simulink model "CCCV_Trial_6"  (R2022b)
settings: Solver=VariableStepAuto  StartTime=0.0  StopTime=3600  RelTol=1e-3
libraries: spsSeriesRLCBranchLib x7, spsCurrentMeasurementLib x2, spsDCVoltageSourceLib x1, spsDiodeLib x1, spsGroundLib x1, spsMosfetLib x1, spsVoltageMeasurementLib x1, sps_lib x1
settings Model: Creator=Haposan  LastModifiedBy=Haposan

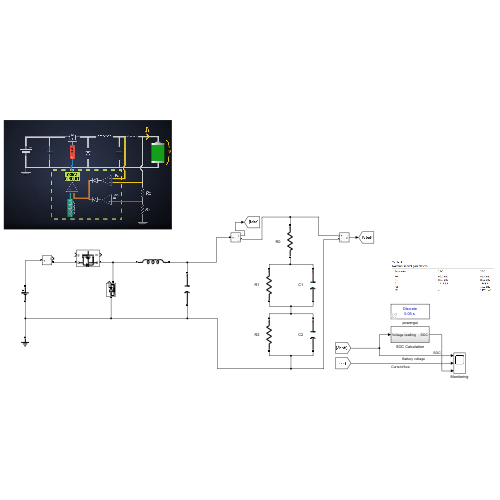
[thumbnail: Simulink's stored preview of the top-level diagram]
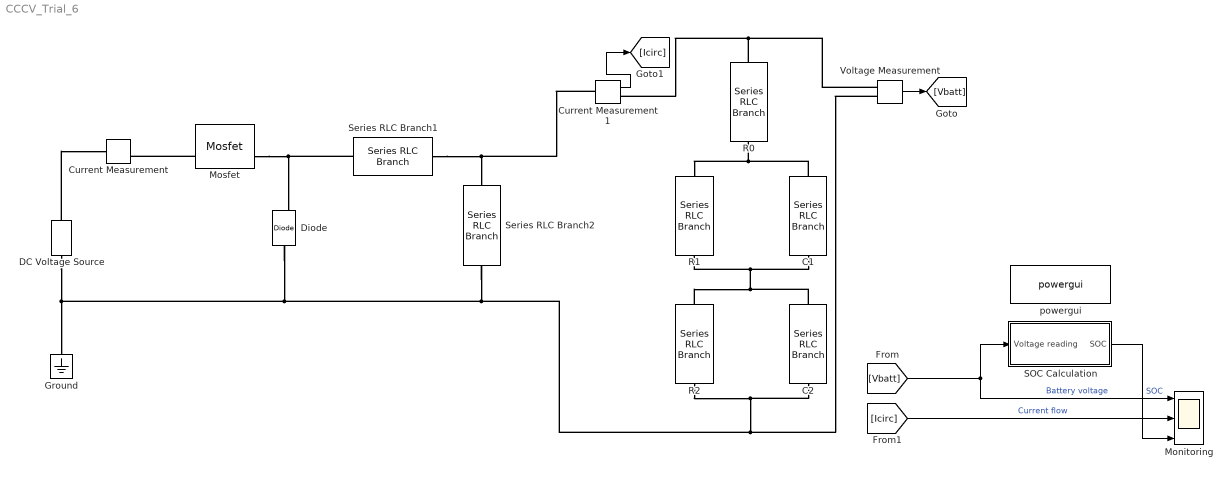
== system CCCV_Trial_6 ==
  C1 : spsSeriesRLCBranchLib/Series RLC Branch  LConnTagsString=__new0  RConnTagsString=__new0  BranchType=C  Resistance=1  Inductance=1e-3  SetiL0=off  InitialCurrent=0  Capacitance=1148  Setx0=off  InitialVoltage=0  Measurements=None
  C2 : spsSeriesRLCBranchLib/Series RLC Branch  LConnTagsString=__new0  RConnTagsString=__new0  BranchType=C  Resistance=1  Inductance=1e-3  SetiL0=off  InitialCurrent=0  Capacitance=117.1e-3  Setx0=off  InitialVoltage=0  Measurements=None
  Current Measurement : spsCurrentMeasurementLib/Current Measurement  PhasorSimulation=off  OutputType=Complex  PSBequivalent=0
  Current Measurement1 : spsCurrentMeasurementLib/Current Measurement  PhasorSimulation=off  OutputType=Complex  PSBequivalent=0
  DC Voltage Source : spsDCVoltageSourceLib/DC Voltage Source  Amplitude=4.2  Measurements=None
  Diode : spsDiodeLib/Diode  Ron=0.001  Lon=0  Vf=0.8  IC=0  UseSnubber=0  Rs=500  Cs=250e-9  Measurements=on
  Ground : spsGroundLib/Ground  LConnTagsString=a
  Monitoring : Scope  NumInputPorts=3
  Mosfet : spsMosfetLib/Mosfet  Ron=0.1  Lon=0  Rd=0.01  Vfd=0  IC=0  Rs=1e5  Cs=inf  Measurements=on
  R0 : spsSeriesRLCBranchLib/Series RLC Branch  LConnTagsString=__new0  RConnTagsString=__new0  BranchType=R  Resistance=56.4e-3  Inductance=1e-3  SetiL0=off  InitialCurrent=0  Capacitance=200e-6  Setx0=off  InitialVoltage=0  Measurements=None
  R1 : spsSeriesRLCBranchLib/Series RLC Branch  LConnTagsString=__new0  RConnTagsString=__new0  BranchType=R  Resistance=35.2e-3  Inductance=1e-3  SetiL0=off  InitialCurrent=0  Capacitance=200e-6  Setx0=off  InitialVoltage=0  Measurements=None
  R2 : spsSeriesRLCBranchLib/Series RLC Branch  LConnTagsString=__new0  RConnTagsString=__new0  BranchType=R  Resistance=13.2e-3  Inductance=1e-3  SetiL0=off  InitialCurrent=0  Capacitance=200e-6  Setx0=off  InitialVoltage=0  Measurements=None
  SOC Calculation : Subsystem
  Series RLC Branch1 : spsSeriesRLCBranchLib/Series RLC Branch  LConnTagsString=__new0  RConnTagsString=__new0  BranchType=L  Resistance=1  Inductance=150e-4  SetiL0=off  InitialCurrent=0  Capacitance=1e-6  Setx0=off  InitialVoltage=0  Measurements=None
  Series RLC Branch2 : spsSeriesRLCBranchLib/Series RLC Branch  LConnTagsString=__new0  RConnTagsString=__new0  BranchType=C  Resistance=1  Inductance=1e-3  SetiL0=off  InitialCurrent=0  Capacitance=1  Setx0=off  InitialVoltage=0  Measurements=None
  Voltage Measurement : spsVoltageMeasurementLib/Voltage Measurement  PhasorSimulation=off  OutputType=Complex  PSBequivalent=0
  powergui : sps_lib/powergui  Priority=1  SimulationMode=Discrete  SampleTime=50e-3  frequency=60  Iterations=50  frequencyindice=0  Pbase=100e6  ErrMax=1e-4  UnitsV=kV  UnitsW=MW  buscounter=0  FunctionMessages=off  echomessages=off  EnableUseOfTLC=off  CurrentSourceSwitches=off  DisableSnubberDevices=off  DisableRonSwitches=off  DisableVfSwitches=off  DisplayEquations=off  AutomaticDiscreteSolvers=off  SolverType=Tustin/Backward Euler (TBE)  Interpol=off  ExternalGateDelay=off  methode=off  Ts=100  x0status=blocks  SPID=on  SwTol=0  HookPort=off  NonlinearTolerance=1e-4  nMaxIteration=100  ContinueOnMaxIteration=off  RestoreLinks=warning  ResistiveCurrentMeasurement=off  Frange=[0:2:500]  Ylog=off  Xlog=on  ShowGrid=off  save=off  variable=ZData  structure=0  ZoomFFT=off  StartTime=0.0  cycles=1  DisplayStyle=1  fundamental=60  FreqAxis=off  MaxFrequency=1000  frequencyindicesteady=1  RmsSteady=1  display=off
  wires:
  SOC Calculation/1(SOC) -> Monitoring/3  "SOC"
  [Icirc] -> Monitoring/2  "Current flow"
  [Vbatt] -> SOC Calculation/1(Voltage reading), Monitoring/1  "Battery voltage"
  Voltage Measurement/1 -> [Vbatt]
  Current Measurement1/1 -> [Icirc]
  connections:
  DC Voltage Source/RConn1 -- Current Measurement/LConn1
  DC Voltage Source/LConn1 -- Voltage Measurement/LConn2 -- C2/RConn1 -- R2/RConn1 -- Series RLC Branch2/RConn1 -- Diode/LConn1 -- Ground/LConn1
  Series RLC Branch1/RConn1 -- Mosfet/RConn1 -- Diode/RConn1
  Series RLC Branch1/LConn1 -- Current Measurement1/LConn1 -- Series RLC Branch2/LConn1
  C1/LConn1 -- R1/LConn1 -- R0/RConn1
  C2/LConn1 -- R2/LConn1 -- C1/RConn1 -- R1/RConn1
  R0/LConn1 -- Voltage Measurement/LConn1 -- Current Measurement1/RConn1
  Mosfet/LConn1 -- Current Measurement/RConn1

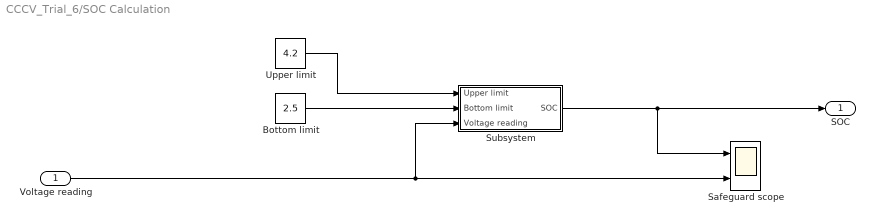
== system CCCV_Trial_6/SOC Calculation ==
  Voltage reading : Inport
  Bottom limit : Constant  Value=2.5
  Safeguard scope : Scope  NumInputPorts=2
  Subsystem : Subsystem
  Upper limit : Constant  Value=4.2
  SOC : Outport
  wires:
  Bottom limit/1 -> Subsystem/2(Bottom limit)
  Voltage reading/1 -> Safeguard scope/2, Subsystem/3(Voltage reading)
  Upper limit/1 -> Subsystem/1(Upper limit)
  Subsystem/1(SOC) -> Safeguard scope/1, SOC/1

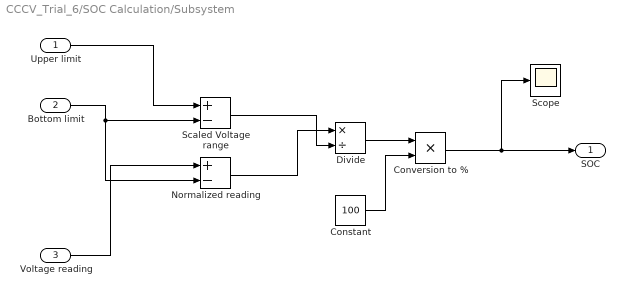
== system CCCV_Trial_6/SOC Calculation/Subsystem ==
  Upper limit : Inport
  Bottom limit : Inport  Port=2
  Voltage reading : Inport  Port=3
  Constant : Constant  Value=100
  Conversion to % : Product
  Divide : Product  Inputs=*/
  Normalized reading : Sum  Inputs=+-
  Scaled Voltage range : Sum  Inputs=+-
  Scope : Scope
  SOC : Outport
  wires:
  Upper limit/1 -> Scaled Voltage range/1
  Bottom limit/1 -> Normalized reading/2, Scaled Voltage range/2
  Voltage reading/1 -> Normalized reading/1
  Normalized reading/1 -> Divide/1
  Scaled Voltage range/1 -> Divide/2
  Divide/1 -> Conversion to %/1
  Constant/1 -> Conversion to %/2
  Conversion to %/1 -> Scope/1, SOC/1
